simulink model "ConfiguredVirtualVehicleModel"  (R2025b)
settings: Solver=ode14x  StartTime=0  StopTime=inf  FixedStep=.001  RelTol=1e-2  EnableMultiTasking=on
StopFcn:
  | %toc
undefined symbols (not defined in the file or in its folder): CtrlTcuInitGear, DriverPreviewDist, EnvAbsPrs, EnvAirTemp, EnvGrvty, EnvNomFrictionScaling, EnvNominalGrade, EnvWindVelX, EnvWindVelY, EnvWindVelZ, MotoFrmInert, MotoFrmLngth, MotoFrmMass, MotoLowrFrntFrkMass, MotoRearArmLngth, MotoRearArmMass, MotoUpprFrntFrkMass, PlntEngTqMax, RiderMass, Sim3dSensor, trackData
libraries: sm_lib x12, simulink x11, nesl_utility x8, sim3dgroundtruthsensorlib x2, autolibshared x2, vehdynlibdriver x2, instrumentseriallib x2, sharedtransform x1, vehdynlibviscommon x1, autolibutils x1, vehdynlibscenariocommon x1, vehdynlibsteering x1
(part 5 of 5)

== system ConfiguredVirtualVehicleModel/Rider Commands/Rider Commands/Roll angle control/Rider Steering Control/Rider Steering/Target trajectory driving - Look ahead point/LAPview ==
  px : Inport
  pz : Inport  Port=2
  Cartesian Joint : sm_lib/Joints/Cartesian Joint  JointMode=Normal  CompositeWrenchDir=FollowerOnBase  CompositeWrenchFrame=BaseFrame  SenseConstraintForce=off  SenseConstraintTorque=off  SenseTotalForce=off  SenseTotalTorque=off  PxPositionTargetSpecify=on  PxPositionTargetPriority=High  PxPositionTargetValue=5  PxPositionTargetValueUnits=m  PxVelocityTargetSpecify=off  PxVelocityTargetPriority=High  PxVelocityTargetValue=0  PxVelocityTargetValueUnits=m/s  PxEquilibriumPosition=0  PxEquilibriumPositionUnits=m  PxSpringStiffness=0  PxSpringStiffnessUnits=N/m  PxDampingCoefficient=0  PxDampingCoefficientUnits=N/(m/s)  PxLowerLimitSpecify=off  PxLowerLimitBound=-1  PxLowerLimitBoundUnits=m  PxLowerLimitStiffness=1e6  PxLowerLimitStiffnessUnits=N/m  PxLowerLimitDamping=1e3  PxLowerLimitDampingUnits=N/(m/s)  PxLowerLimitTransitionRegionWidth=1e-4  PxLowerLimitTransitionRegionWidthUnits=m  PxUpperLimitSpecify=off  PxUpperLimitBound=1  PxUpperLimitBoundUnits=m  PxUpperLimitStiffness=1e6  PxUpperLimitStiffnessUnits=N/m  PxUpperLimitDamping=1e3  PxUpperLimitDampingUnits=N/(m/s)  PxUpperLimitTransitionRegionWidth=1e-4  PxUpperLimitTransitionRegionWidthUnits=m  PxTorqueActuationMode=ComputedTorque  PxMotionActuationMode=InputMotion  PxSensePosition=off  PxSenseVelocity=off  PxSenseAcceleration=off  PxSenseTorqueForce=off  PxSenseLowerLimitTorqueForce=off  PxSenseUpperLimitTorqueForce=off  PyPositionTargetSpecify=off  PyPositionTargetPriority=High  PyPositionTargetValue=0  PyPositionTargetValueUnits=m  PyVelocityTargetSpecify=off  PyVelocityTargetPriority=High  PyVelocityTargetValue=0  PyVelocityTargetValueUnits=m/s  PyEquilibriumPosition=0  PyEquilibriumPositionUnits=m  PySpringStiffness=0  PySpringStiffnessUnits=N/m  PyDampingCoefficient=0  PyDampingCoefficientUnits=N/(m/s)  PyLowerLimitSpecify=off  PyLowerLimitBound=-1  PyLowerLimitBoundUnits=m  PyLowerLimitStiffness=1e6  PyLowerLimitStiffnessUnits=N/m  PyLowerLimitDamping=1e3  PyLowerLimitDampingUnits=N/(m/s)  PyLowerLimitTransitionRegionWidth=1e-4  PyLowerLimitTransitionRegionWidthUnits=m  PyUpperLimitSpecify=off  PyUpperLimitBound=1  PyUpperLimitBoundUnits=m  PyUpperLimitStiffness=1e6  PyUpperLimitStiffnessUnits=N/m  PyUpperLimitDamping=1e3  PyUpperLimitDampingUnits=N/(m/s)  PyUpperLimitTransitionRegionWidth=1e-4  PyUpperLimitTransitionRegionWidthUnits=m  PyTorqueActuationMode=ComputedTorque  PyMotionActuationMode=InputMotion  PySensePosition=off  PySenseVelocity=off  PySenseAcceleration=off  PySenseTorqueForce=off  PySenseLowerLimitTorqueForce=off  PySenseUpperLimitTorqueForce=off  PzPositionTargetSpecify=off  PzPositionTargetPriority=High  PzPositionTargetValue=0  PzPositionTargetValueUnits=m  PzVelocityTargetSpecify=off  PzVelocityTargetPriority=High  PzVelocityTargetValue=0  PzVelocityTargetValueUnits=m/s  PzEquilibriumPosition=0  PzEquilibriumPositionUnits=m  PzSpringStiffness=0  PzSpringStiffnessUnits=N/m  PzDampingCoefficient=0  PzDampingCoefficientUnits=N/(m/s)  PzLowerLimitSpecify=off  PzLowerLimitBound=-1  PzLowerLimitBoundUnits=m  PzLowerLimitStiffness=1e6  PzLowerLimitStiffnessUnits=N/m  PzLowerLimitDamping=1e3  PzLowerLimitDampingUnits=N/(m/s)  PzLowerLimitTransitionRegionWidth=1e-4  PzLowerLimitTransitionRegionWidthUnits=m  PzUpperLimitSpecify=off  PzUpperLimitBound=1  PzUpperLimitBoundUnits=m  PzUpperLimitStiffness=1e6  PzUpperLimitStiffnessUnits=N/m  PzUpperLimitDamping=1e3  PzUpperLimitDampingUnits=N/(m/s)  PzUpperLimitTransitionRegionWidth=1e-4  PzUpperLimitTransitionRegionWidthUnits=m  PzTorqueActuationMode=ComputedTorque  PzMotionActuationMode=InputMotion  PzSensePosition=off  PzSenseVelocity=off  PzSenseAcceleration=off  PzSenseTorqueForce=off  PzSenseLowerLimitTorqueForce=off  PzSenseUpperLimitTorqueForce=off
  Constant : Constant  Value=0
  Origin&Env : Subsystem
  Simulink-PS Converter : nesl_utility/Simulink-PS Converter  PhysicalDomain=network_engine_domain  SubClassName=ps_input  LeftPortType=input  RightPortType=output  PseudoPeriodic=off  Frequencies=[]  NoiseDistribution=none  NoiseParameters=[]  Unit=1  AffineConversion=off  FilteringAndDerivatives=filter  SimscapeFilterOrder=2  InputFilterTimeConstant=0.001  UdotUserProvided=0
  Simulink-PS Converter1 : nesl_utility/Simulink-PS Converter  PhysicalDomain=network_engine_domain  SubClassName=ps_input  LeftPortType=input  RightPortType=output  PseudoPeriodic=off  Frequencies=[]  NoiseDistribution=none  NoiseParameters=[]  Unit=1  AffineConversion=off  FilteringAndDerivatives=filter  SimscapeFilterOrder=2  InputFilterTimeConstant=0.001  UdotUserProvided=0
  Simulink-PS Converter2 : nesl_utility/Simulink-PS Converter  PhysicalDomain=network_engine_domain  SubClassName=ps_input  LeftPortType=input  RightPortType=output  PseudoPeriodic=off  Frequencies=[]  NoiseDistribution=none  NoiseParameters=[]  Unit=1  AffineConversion=off  FilteringAndDerivatives=filter  SimscapeFilterOrder=2  InputFilterTimeConstant=0.001  UdotUserProvided=0
  Spherical Solid : sm_lib/Body Elements/Spherical Solid  SphereRadius=0.1  SphereRadiusUnits=m  ExportEntireGeometry=off  InertiaType=CalculateFromGeometry  BasedOnType=Density  Density=1000  DensityUnits=kg/m^3  Mass=1  MassUnits=kg  CenterOfMass=[0 0 0]  CenterOfMassUnits=m  MomentsOfInertia=[1 1 1]  MomentsOfInertiaUnits=kg*m^2  ProductsOfInertia=[0 0 0]  ProductsOfInertiaUnits=kg*m^2  GraphicType=FromGeometry  MarkerShape=Sphere  MarkerSize=10  GraphicVisPropType=SimpleVisualProperties  GraphicDiffuseColor=[1.0 0.2 0.2]  GraphicOpacity=1.0  GraphicSpecularColor=[0.5 0.5 0.5 1.0]  GraphicAmbientColor=[0.15 0.15 0.15 1.0]  GraphicEmissiveColor=[0.0 0.0 0.0 1.0]  GraphicShininess=75  DoExposeReferenceFrame=on  SerializedFrames=<Frames/>
  wires:
  pz/1 -> Simulink-PS Converter1/1
  px/1 -> Simulink-PS Converter/1
  Constant/1 -> Simulink-PS Converter2/1
  connections:
  Simulink-PS Converter2/RConn1 -- Cartesian Joint/LConn4
  Spherical Solid/RConn1 -- Cartesian Joint/RConn1
  Simulink-PS Converter/RConn1 -- Cartesian Joint/LConn2
  Cartesian Joint/LConn1 -- Origin&Env/LConn1
  Simulink-PS Converter1/RConn1 -- Cartesian Joint/LConn3

== system ConfiguredVirtualVehicleModel/Rider Commands/Rider Commands/Roll angle control/Rider Steering Control/Rider Steering/Target trajectory driving - Look ahead point/feedback ==
  note: derive target roll angle
  mindist : Inport
  roll : Inport  Port=2
  rollRate : Inport  Port=3
  Gain1 : Gain  Gain=RidTrajContG
  KphiRM : Gain  Gain=RidTrajContGphi
  KphidRM : Gain  Gain=RidTrajContGphid
  Sum : Sum  Inputs=|+-
  Sum1 : Sum  Inputs=|++
  control torque : Outport  VectorParamsAs1DForOutWhenUnconnected=off
  wires:
  roll/1 -> Sum/2
  Gain1/1 -> Sum/1
  rollRate/1 -> KphidRM/1
  KphiRM/1 -> Sum1/1
  KphidRM/1 -> Sum1/2
  Sum/1 -> KphiRM/1
  mindist/1 -> Gain1/1  "mindist"
  Sum1/1 -> control torque/1

== system ConfiguredVirtualVehicleModel/Rider Commands/Rider Commands/Longitudinal Rider/Rider Steering Control/Rider Steering/Target trajectory driving - Look ahead point/LAPview/Origin&Env ==
  Ground : Subsystem
  Mechanism Configuration : sm_lib/Utilities/Mechanism Configuration  UniformGravity=Constant  GravityVector=[0 0 0]  GravityVectorUnits=m/s^2  LinearizationDelta=0.001  JointModeTransitionNonlinearIterations=2
  Solver Configuration : nesl_utility/Solver Configuration  PhysicalDomain=network_engine_domain  SubClassName=solver  LeftPortType=input  RightPortType=generic  Tones=[]  Harmonics=[]  SimulateNoise=off  Profile=off  UseLocalSampling=off  EnableSwitchedLinearOptims=on  FrequencyDomain=off  UseCCode=off  RelTol=0.001  AbsTol=1e-06  MinStep=1e-09  ToWorkspace=off  RevertToSquareIcSolve=off  NumHomotopyIterations=100  PhasorMode=off  PhasorModeNumHarmonics=1  ConsistencySolver=NEWTON_FTOL  IndexReductionMethod=DerivativeReplacement  DoDC=off  ResidualTolerance=1e-09  ConsistencyTolSource=GLOBAL  ConsistencyAbsTol=0.001  ConsistencyRelTol=0.001  ConsistencyTolFactor=0.001  UseLocalSolver=off  LocalSolverChoice=NE_BACKWARD_EULER_ADVANCER  ResolveIndetEquations=on  FunctionEvalNumThread=1  LocalSolverSampleTime=0.001  DoFixedCost=off  MaxNonlinIter=3  MaxModeIter=2  ComputeImpulses=off  ImpulseIterations=2  LinearAlgebra=Sparse  LinearAlgebraNumThread=0  EquationFormulation=NE_TIME_EF  DelaysMemoryBudget=1024  AutomaticFiltering=on  FilteringTimeConstant=0.001  PartitionStorageMethod=AS_NEEDED  PartitionMemoryBudget=1024  PartitionMethod=FAST  MultibodyUseLocalSolver=off  MultibodyLocalSolverChoice=ODE1  MultibodyLocalSolverSampleTime=0.001
  World Frame : sm_lib/Frames and Transforms/World Frame
  F : PMIOPort  Side=Left
  connections:
  World Frame/RConn1 -- Ground/LConn1 -- F/RConn1 -- Mechanism Configuration/RConn1 -- Solver Configuration/RConn1

== system ConfiguredVirtualVehicleModel/Rider Commands/Rider Commands/Roll angle control/Rider Steering Control/Rider Steering/Target trajectory driving - Look ahead point/LAPview/Origin&Env ==
  Ground : Subsystem
  Mechanism Configuration : sm_lib/Utilities/Mechanism Configuration  UniformGravity=Constant  GravityVector=[0 0 0]  GravityVectorUnits=m/s^2  LinearizationDelta=0.001  JointModeTransitionNonlinearIterations=2
  Solver Configuration : nesl_utility/Solver Configuration  PhysicalDomain=network_engine_domain  SubClassName=solver  LeftPortType=input  RightPortType=generic  Tones=[]  Harmonics=[]  SimulateNoise=off  Profile=off  UseLocalSampling=off  EnableSwitchedLinearOptims=on  FrequencyDomain=off  UseCCode=off  RelTol=0.001  AbsTol=1e-06  MinStep=1e-09  ToWorkspace=off  RevertToSquareIcSolve=off  NumHomotopyIterations=100  PhasorMode=off  PhasorModeNumHarmonics=1  ConsistencySolver=NEWTON_FTOL  IndexReductionMethod=DerivativeReplacement  DoDC=off  ResidualTolerance=1e-09  ConsistencyTolSource=GLOBAL  ConsistencyAbsTol=0.001  ConsistencyRelTol=0.001  ConsistencyTolFactor=0.001  UseLocalSolver=off  LocalSolverChoice=NE_BACKWARD_EULER_ADVANCER  ResolveIndetEquations=on  FunctionEvalNumThread=1  LocalSolverSampleTime=0.001  DoFixedCost=off  MaxNonlinIter=3  MaxModeIter=2  ComputeImpulses=off  ImpulseIterations=2  LinearAlgebra=Sparse  LinearAlgebraNumThread=0  EquationFormulation=NE_TIME_EF  DelaysMemoryBudget=1024  AutomaticFiltering=on  FilteringTimeConstant=0.001  PartitionStorageMethod=AS_NEEDED  PartitionMemoryBudget=1024  PartitionMethod=FAST  MultibodyUseLocalSolver=off  MultibodyLocalSolverChoice=ODE1  MultibodyLocalSolverSampleTime=0.001
  World Frame : sm_lib/Frames and Transforms/World Frame
  F : PMIOPort  Side=Left
  connections:
  World Frame/RConn1 -- Ground/LConn1 -- F/RConn1 -- Mechanism Configuration/RConn1 -- Solver Configuration/RConn1

== system ConfiguredVirtualVehicleModel/Rider Commands/Rider Commands/Longitudinal Rider/Rider Steering Control/Rider Steering/Target trajectory driving - Look ahead point/LAPview/Origin&Env/Ground ==
  Spline : sm_lib/Curves and Surfaces/Spline  DataPoints=trackData'+[0 0 0.001]  DataPointsUnits=m  EndConditionType=Natural  GraphicType=FromGeometry  MarkerShape=Sphere  MarkerSize=10  GraphicVisPropType=SimpleVisualProperties  GraphicDiffuseColor=[0.2 1.0 1.0]  GraphicOpacity=1.0  GraphicSpecularColor=[0.5 0.5 0.5 1.0]  GraphicAmbientColor=[0.15 0.15 0.15 1.0]  GraphicEmissiveColor=[0.0 0.0 0.0 1.0]  GraphicShininess=75
  Weld Joint : sm_lib/Joints/Weld Joint  JointMode=Normal  CompositeWrenchDir=FollowerOnBase  CompositeWrenchFrame=BaseFrame  SenseConstraintForce=off  SenseConstraintTorque=off  SenseTotalForce=off  SenseTotalTorque=off
  B : PMIOPort  Side=Left
  connections:
  Weld Joint/LConn1 -- B/RConn1
  Spline/LConn1 -- Weld Joint/RConn1

== system ConfiguredVirtualVehicleModel/Rider Commands/Rider Commands/Roll angle control/Rider Steering Control/Rider Steering/Target trajectory driving - Look ahead point/LAPview/Origin&Env/Ground ==
  Spline : sm_lib/Curves and Surfaces/Spline  DataPoints=trackData'+[0 0 0.001]  DataPointsUnits=m  EndConditionType=Natural  GraphicType=FromGeometry  MarkerShape=Sphere  MarkerSize=10  GraphicVisPropType=SimpleVisualProperties  GraphicDiffuseColor=[0.2 1.0 1.0]  GraphicOpacity=1.0  GraphicSpecularColor=[0.5 0.5 0.5 1.0]  GraphicAmbientColor=[0.15 0.15 0.15 1.0]  GraphicEmissiveColor=[0.0 0.0 0.0 1.0]  GraphicShininess=75
  Weld Joint : sm_lib/Joints/Weld Joint  JointMode=Normal  CompositeWrenchDir=FollowerOnBase  CompositeWrenchFrame=BaseFrame  SenseConstraintForce=off  SenseConstraintTorque=off  SenseTotalForce=off  SenseTotalTorque=off
  B : PMIOPort  Side=Left
  connections:
  Weld Joint/LConn1 -- B/RConn1
  Spline/LConn1 -- Weld Joint/RConn1

== matlab function ConfiguredVirtualVehicleModel/Rider Commands/Rider Commands/Longitudinal Rider/Rider Steering Control/Rider Steering/Target trajectory driving - Look ahead point/LateralDeviationDeriver ==
  settings: updateMethod=DISCRETE  sampleTime=1e-2
  data: current_x input; mindist_out output; current_y input; VehicleYaw input; trackData parameter
%%%%%%%%%%%%%%%%%%%%%%%%%%%%%%%%%%%%%%%%%%%%%%%%%%%%%%%%%%%%%%%%%%%%%%%%%%%
%                      Lateral Deviation Deriver
%
% This script derive lateral distance between lookahead point and target
% path
%%%%%%%%%%%%%%%%%%%%%%%%%%%%%%%%%%%%%%%%%%%%%%%%%%%%%%%%%%%%%%%%%%%%%%%%%%%
function mindist_out =  LateralDeviationDeriver(current_x, current_y, VehicleYaw, trackData)

mindist_out =  LateralDeviationDeriver_s(trackData, current_x, current_y, VehicleYaw);

if isnan(mindist_out)
    disp('nan!!!');
end

end

function mindist_out =  LateralDeviationDeriver_s(Target, current_x, current_y, VehicleYaw)

coder.allowpcode('plain');

% Tick = 0.1;
% 
%-------------------------------------------------------------------------%
% TARGET PATH
%-------------------------------------------------------------------------%
Target_X = Target(1,:);
Target_Y = Target(2,:);

% % interpolate
% tmp_elem     = 1:length(tmp_Target_X);
% tmp_elem_int = 1:Tick:length(tmp_Target_X);
% Target_X = interp1(tmp_elem, tmp_Target_X, tmp_elem_int,'spline');
% Target_Y = interp1(tmp_elem, tmp_Target_Y, tmp_elem_int,'spline');

%-------------------------------------------------------------------------%
% ROTATION
%-------------------------------------------------------------------------%
% rotation matrix
rotmat_yaw = [cos(VehicleYaw), -sin(VehicleYaw); sin(VehicleYaw), cos(VehicleYaw)];

% rotate target path
tmp_Target  = transpose(rotmat_yaw) * [Target_X; Target_Y];
Target_Xrot = tmp_Target(1,:);
Target_Yrot = tmp_Target(2,:);

% rotate current position
tmp_current  = transpose(rotmat_yaw) * [current_x; current_y];
current_xrot = tmp_current(1,:);
current_yrot = tmp_current(2,:);

% distance between LAP and all points
dist = sqrt((current_xrot - Target_Xrot).^2 + (current_yrot - Target_Yrot).^2);

% minimum distance point
[~, col]      = find(dist == min(abs(dist)));
% point_out = Target_Xrot(col);

%
if col(end) < length(Target_Xrot)
theta = atan((Target_Yrot(col(end)+1) - Target_Yrot(col(end))) / (Target_Xrot(col(end)+1) - Target_Xrot(col(end)))); % ??????????
else
theta = atan((Target_Yrot(col(end)) - Target_Yrot(col(end)-1)) / (Target_Xrot(col(end)) - Target_Xrot(col(end)-1)));
end

% rotation matrix
rotmat = [cos(theta), -sin(theta); sin(theta), cos(theta)];

% Coordinate transformation
if col(end) < length(Target_Xrot)
ABC_XY = [Target_Xrot(col(end)), Target_Xrot(col(end)+1), current_xrot; Target_Yrot(col(end)), Target_Yrot(col(end)+1), current_yrot];
else
ABC_XY = [Target_Xrot(col(end)-1), Target_Xrot(col(end)), current_xrot; Target_Yrot(col(end)-1), Target_Yrot(col(end)), current_yrot];
end
ABC_XYrot = transpose(rotmat) * ABC_XY;

% area
A_x = ABC_XYrot(1,1);
B_x = ABC_XYrot(1,2);
C_x = ABC_XYrot(1,3);
C_y = ABC_XYrot(2,3)-ABC_XYrot(2,1);

    area_out = 0;
if A_x <= C_x && C_x <= B_x
    area_out = 0;
elseif  C_x < A_x
    area_out = -1;
elseif  B_x < C_x
    area_out = 1;
end

% area
if area_out == -1
    if col(end) ~= 1
        if Target_Xrot(col(end)) ~= Target_Xrot(col(end)-1)
            theta = atan((Target_Yrot(col(end)) - Target_Yrot(col(end)-1)) / (Target_Xrot(col(end)) - Target_Xrot(col(end)-1)));
        else
            theta = 0;
        end
rotmat = [cos(theta), -sin(theta); sin(theta), cos(theta)];

ABC_XY = [Target_Xrot(col(end)-1), Target_Xrot(col(end)), current_xrot; Target_Yrot(col(end)-1), Target_Yrot(col(end)), current_yrot];
    else
        if Target_Xrot(col(end)) ~= Target_Xrot(end)
            theta = atan((Target_Yrot(col(end)) - Target_Yrot(end)) / (Target_Xrot(col(end)) - Target_Xrot(end)));
        else
            theta = 0;
        end
rotmat = [cos(theta), -sin(theta); sin(theta), cos(theta)];

ABC_XY = [Target_Xrot(end), Target_Xrot(col(end)), current_xrot; Target_Yrot(end), Target_Yrot(col(end)), current_yrot];
    end
    
ABC_XYrot = transpose(rotmat) * ABC_XY;

% A.y = ABC_XYrot(2,1);
% B.y = ABC_XYrot(2,2);
C_y = ABC_XYrot(2,3)-ABC_XYrot(2,1);
end

% minimum distance
mindist_out = C_y;
end

== matlab function ConfiguredVirtualVehicleModel/Rider Commands/Rider Commands/Roll angle control/Rider Steering Control/Rider Steering/Target trajectory driving - Look ahead point/LateralDeviationDeriver ==
  settings: updateMethod=DISCRETE  sampleTime=1e-2
  data: current_x input; mindist_out output; current_y input; VehicleYaw input; trackData parameter
%%%%%%%%%%%%%%%%%%%%%%%%%%%%%%%%%%%%%%%%%%%%%%%%%%%%%%%%%%%%%%%%%%%%%%%%%%%
%                      Lateral Deviation Deriver
%
% This script derive lateral distance between lookahead point and target
% path
%%%%%%%%%%%%%%%%%%%%%%%%%%%%%%%%%%%%%%%%%%%%%%%%%%%%%%%%%%%%%%%%%%%%%%%%%%%
function mindist_out =  LateralDeviationDeriver(current_x, current_y, VehicleYaw, trackData)

mindist_out =  LateralDeviationDeriver_s(trackData, current_x, current_y, VehicleYaw);

if isnan(mindist_out)
    disp('nan!!!');
end

end

function mindist_out =  LateralDeviationDeriver_s(Target, current_x, current_y, VehicleYaw)

coder.allowpcode('plain');

% Tick = 0.1;
% 
%-------------------------------------------------------------------------%
% TARGET PATH
%-------------------------------------------------------------------------%
Target_X = Target(1,:);
Target_Y = Target(2,:);

% % interpolate
% tmp_elem     = 1:length(tmp_Target_X);
% tmp_elem_int = 1:Tick:length(tmp_Target_X);
% Target_X = interp1(tmp_elem, tmp_Target_X, tmp_elem_int,'spline');
% Target_Y = interp1(tmp_elem, tmp_Target_Y, tmp_elem_int,'spline');

%-------------------------------------------------------------------------%
% ROTATION
%-------------------------------------------------------------------------%
% rotation matrix
rotmat_yaw = [cos(VehicleYaw), -sin(VehicleYaw); sin(VehicleYaw), cos(VehicleYaw)];

% rotate target path
tmp_Target  = transpose(rotmat_yaw) * [Target_X; Target_Y];
Target_Xrot = tmp_Target(1,:);
Target_Yrot = tmp_Target(2,:);

% rotate current position
tmp_current  = transpose(rotmat_yaw) * [current_x; current_y];
current_xrot = tmp_current(1,:);
current_yrot = tmp_current(2,:);

% distance between LAP and all points
dist = sqrt((current_xrot - Target_Xrot).^2 + (current_yrot - Target_Yrot).^2);

% minimum distance point
[~, col]      = find(dist == min(abs(dist)));
% point_out = Target_Xrot(col);

%
if col(end) < length(Target_Xrot)
theta = atan((Target_Yrot(col(end)+1) - Target_Yrot(col(end))) / (Target_Xrot(col(end)+1) - Target_Xrot(col(end)))); % ??????????
else
theta = atan((Target_Yrot(col(end)) - Target_Yrot(col(end)-1)) / (Target_Xrot(col(end)) - Target_Xrot(col(end)-1)));
end

% rotation matrix
rotmat = [cos(theta), -sin(theta); sin(theta), cos(theta)];

% Coordinate transformation
if col(end) < length(Target_Xrot)
ABC_XY = [Target_Xrot(col(end)), Target_Xrot(col(end)+1), current_xrot; Target_Yrot(col(end)), Target_Yrot(col(end)+1), current_yrot];
else
ABC_XY = [Target_Xrot(col(end)-1), Target_Xrot(col(end)), current_xrot; Target_Yrot(col(end)-1), Target_Yrot(col(end)), current_yrot];
end
ABC_XYrot = transpose(rotmat) * ABC_XY;

% area
A_x = ABC_XYrot(1,1);
B_x = ABC_XYrot(1,2);
C_x = ABC_XYrot(1,3);
C_y = ABC_XYrot(2,3)-ABC_XYrot(2,1);

    area_out = 0;
if A_x <= C_x && C_x <= B_x
    area_out = 0;
elseif  C_x < A_x
    area_out = -1;
elseif  B_x < C_x
    area_out = 1;
end

% area
if area_out == -1
    if col(end) ~= 1
        if Target_Xrot(col(end)) ~= Target_Xrot(col(end)-1)
            theta = atan((Target_Yrot(col(end)) - Target_Yrot(col(end)-1)) / (Target_Xrot(col(end)) - Target_Xrot(col(end)-1)));
        else
            theta = 0;
        end
rotmat = [cos(theta), -sin(theta); sin(theta), cos(theta)];

ABC_XY = [Target_Xrot(col(end)-1), Target_Xrot(col(end)), current_xrot; Target_Yrot(col(end)-1), Target_Yrot(col(end)), current_yrot];
    else
        if Target_Xrot(col(end)) ~= Target_Xrot(end)
            theta = atan((Target_Yrot(col(end)) - Target_Yrot(end)) / (Target_Xrot(col(end)) - Target_Xrot(end)));
        else
            theta = 0;
        end
rotmat = [cos(theta), -sin(theta); sin(theta), cos(theta)];

ABC_XY = [Target_Xrot(end), Target_Xrot(col(end)), current_xrot; Target_Yrot(end), Target_Yrot(col(end)), current_yrot];
    end
    
ABC_XYrot = transpose(rotmat) * ABC_XY;

% A.y = ABC_XYrot(2,1);
% B.y = ABC_XYrot(2,2);
C_y = ABC_XYrot(2,3)-ABC_XYrot(2,1);
end

% minimum distance
mindist_out = C_y;
end

== matlab function ConfiguredVirtualVehicleModel/Visualization/Excessive Roll Angle Detection ==
  data: phi input; stopSim output
function stopSim = phiStop(phi)
%#codegen

% Initialize output
stopSim = false;

% Check the condition
rollLim = pi/3;
if abs(phi)>=rollLim
    % Display a warning message    
    warning(message('vdynblks:vehdynErrMsg:excessivePhi',num2str(rad2deg(rollLim))));
    % Set output to indicate a warning has been triggered
    stopSim = true;
end

== matlab function ConfiguredVirtualVehicleModel/Server Communication/UDPSend ==
  data: engspeed input; angspeed input; temp input; emissions input; fuel input; HONK input
function sendData(engspeed, angspeed, temp, emissions, fuel, HONK)
    % 1. TELL SIMULINK TO USE MATLAB ENGINE (Fixes the Code Gen Error)
    coder.extrinsic('udpport', 'write', 'sprintf', 'pi');
    
    % persistent variable to keep the UDP object open between steps
    persistent udpsend;
    
    % 2. INITIALIZE THE PORT
    if isempty(udpsend) 
        % LocalPort 5006 sends TO the Java Server on 5005
        udpsend = udpport("LocalPort", 5006); 
    end
    
    % 3. CALCULATE RPM
    % Using 9.5493 as the conversion factor (60 / 2*pi)
    rpm = angspeed * 9.5493;
    
    % 4. FORMAT THE BIG STRING
    % Example output: "5500.00,85.50,92.10,0.04"
    dataString = sprintf('%.2f,%.2f,%.2f,%.2f,%.2f,%d', rpm, engspeed, temp, emissions, fuel, HONK);
    
    % 5. SEND TO JAVA
    % "char" ensures Java reads standard ASCII/UTF-8 bytes
    write(udpsend, dataString, "char", "127.0.0.1", 5005);
    
end

== matlab function ConfiguredVirtualVehicleModel/Serial Receive/Decode ==
  data: rawByte input; Accel output; Decel output; Gear output; HONK output
function [Accel, Decel, Gear, HONK] = decode(rawByte)
%#codegen

% 1. Isolate the first 6 bits
sixBitValue = bitand(rawByte, uint8(63));

% 2. Extract Accel and Decel (Bits 1 and 2)
% bitget returns 1 or 0. We cast to double for Simulink math compatibility.
Accel = 1- double(bitget(rawByte, 7)); 
Decel = 1-double(bitget(sixBitValue, 2));
HONK = 1-double(bitget(sixBitValue, 3));

% 3. Extract the last 3 bits (Bits 4, 5, 6) for Gear
% Mask with 56 (00111000) and shift right by 3
tempGear = bitand(sixBitValue, uint8(56));
Gear = double(bitsrl(tempGear, 3)); 

% Note: Bit 3 is currently unused in this logic.
end
